simulink model "Mfunction"  (R2020b)
settings: Solver=FixedStepAuto  StartTime=0.0  StopTime=30  RelTol=1e-3
libraries: simulink x1
settings Model: Creator=cesar  LastModifiedBy=cesar

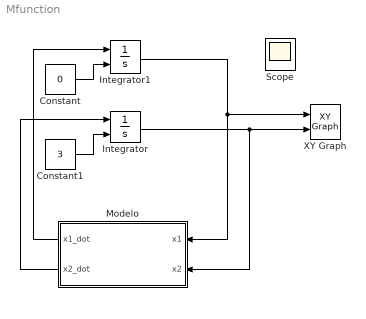
== system Mfunction ==
  Constant : Constant  Value=0
  Constant1 : Constant  Value=3
  Integrator : Integrator  InitialConditionSource=external
  Integrator1 : Integrator  InitialConditionSource=external
  Modelo : MATLAB Function  TreatAsAtomicUnit=on
  Scope : Scope
  XY Graph : simulink/Sinks/XY Graph  xmin=-3  xmax=3  ymin=-3  ymax=3  st=-1
  wires:
  Modelo/1(x1_dot) -> Integrator1/1
  Modelo/2(x2_dot) -> Integrator/1
  Integrator1/1 -> Modelo/1(x1), XY Graph/1
  Integrator/1 -> Modelo/2(x2), XY Graph/2
  Constant1/1 -> Integrator/2
  Constant/1 -> Integrator1/2

== matlab function Mfunction/Modelo ==
  data: x1 input; x1_dot output; x2 input; x2_dot output
function [x1_dot, x2_dot] = fcn(x1, x2)

x1_dot = x2;
x2_dot = -x1 + (1 - x1^2)*x2;
